simulink model "DCDC_SEPIC_ThermalModel"  (R2021b)
settings: Solver=VariableStepAuto  StartTime=0.0  StopTime=3600*24  RelTol=1e-3  EnableMultiTasking=on
undefined symbols (not defined in the file): Curr_Test_Load, Voltage_Test_Vector
libraries: fl_lib x19, nesl_utility x3
Description:
  | Buck Converter Thermal Model
settings Model: FPTRunName=Active  Creator=The MathWorks, Inc.  LastModifiedBy=vlenzi
settings SolverCC: AlgebraicLoopSolver=TrustRegion
settings DataIOCC: MaxDataPoints=10000  SaveFormat=Array  SaveOutput=off  SignalLogging=off  DSMLogging=off  SaveTime=off  SignalLoggingName=logsout_ee_switching_power_supply_thermal_only
settings OptimizationCC: BooleanDataType=off  ExpressionDepthLimit=2147483647  InitFltsAndDblsToZero=on  LifeSpan=1  EfficientTunableParamExpr=on
settings DebuggingCC: SaveWithParameterizedLinksMsg=none  SignalResolutionControl=TryResolveAllWithWarning  MultiTaskDSMMsg=warning  MultiTaskCondExecSysMsg=none  IntegerOverflowMsg=none  ParameterPrecisionLossMsg=none  StateNameClashWarn=warning  SFUnexpectedBacktrackingDiag=warning  SFNoUnconditionalDefaultTransitionDiag=warning  SFExecutionAtInitializationDiag=none  SFMachineParentedDataDiag=warning  IntegerSaturationMsg=none  ArithmeticOperatorsInVariantConditions=warning
settings HardwareCC: ProdBitPerPointer=32  ProdBitPerSizeT=32  ProdBitPerPtrDiffT=32  ProdLargestAtomicFloat=None  ProdIntDivRoundTo=Undefined  ProdEndianess=Unspecified  ProdWordSize=32  ProdHWDeviceType=32-bit Generic
settings ModelReferenceCC: PropagateSignalLabelsOutOfModel=off
settings SFSimCC: SimUseLocalCustomCode=off  CustomCodeUndefinedFunction=UseInterfaceOnly
settings RTWCC: Description=Real-Time Workshop Embedded Coder (no auto configuration)  SystemTargetFile=ert.tlc  TemplateMakefile=ert_default_tmf  GenerateReport=on  RTWUseLocalCustomCode=off  IncludeHyperlinkInReport=on  LaunchReport=on  CreateSILPILBlock=SIL
settings CodeAppCC: IgnoreCustomStorageClasses=off  CustomSymbolStrType=$N$R$M  CustomSymbolStrModelFcn=$N  StateflowObjectComments=on  InternalIdentifier=Classic
settings ERTTargetCC: TargetFcnLib=ansi_tfl_tmw.mat  MultiwordLength=2048  GenerateSampleERTMain=on  ERTCustomFileTemplate=example_file_process.tlc  ConvertIfToSwitch=off  SuppressUnreachableDefaultCases=off
settings ConfigComp: CovMetricSettings=dw  CovSaveCumulativeToWorkspaceVar=on  CovSaveSingleToWorkspaceVar=on  CovExternalEMLEnable=off  CovSFcnEnable=off
settings SimscapeCC: SimscapeLogType=all  SimscapeLogSimulationStatistics=on  SimscapeLogToSDI=on  SimscapeLogName=simlog_ee_switching_power_supply_thermal_only  SimscapeLogLimitData=off  SimscapeLogDataHistory=10000

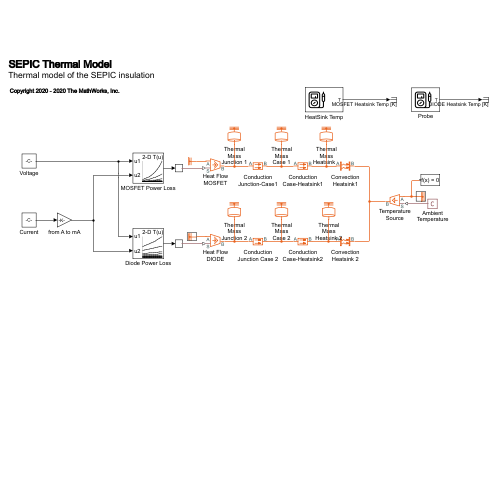
[thumbnail: Simulink's stored preview of the top-level diagram]
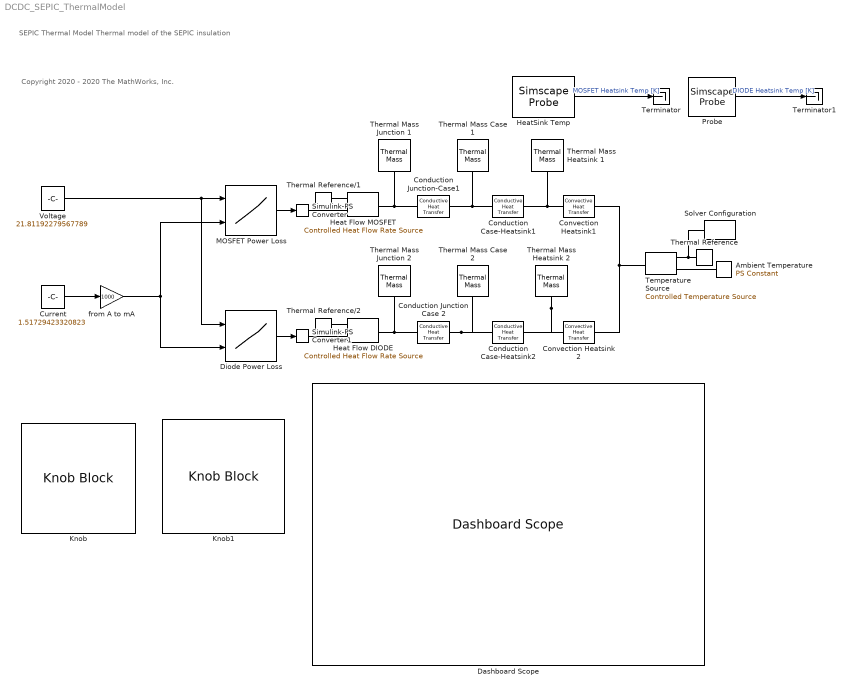
== system DCDC_SEPIC_ThermalModel ==
  note: SEPIC Thermal Model
      | Thermal model of the SEPIC insulation
  note: Copyright 2020 - 2020 The MathWorks, Inc.
  Ambient Temperature : fl_lib/Physical Signals/Sources/PS Constant  constant=298.15
  Conduction Case-Heatsink1 : fl_lib/Thermal/Thermal Elements/Conductive Heat Transfer  area=14 mm^2  thickness=0.1 mm  th_cond=3 W/(m*K)  T_specify=off  T_priority=High  T=0 K  T_nominal_specify=off  T_nominal_unit=K  T_nominal_value=1  Q_specify=off  Q_priority=High  Q=0 J/s  Q_nominal_specify=off  Q_nominal_unit=J/s  Q_nominal_value=1
  Conduction Case-Heatsink2 : fl_lib/Thermal/Thermal Elements/Conductive Heat Transfer  area=14 mm^2  thickness=0.1 mm  th_cond=3 W/(m*K)  T_specify=off  T_priority=High  T=0 K  T_nominal_specify=off  T_nominal_unit=K  T_nominal_value=1  Q_specify=off  Q_priority=High  Q=0 J/s  Q_nominal_specify=off  Q_nominal_unit=J/s  Q_nominal_value=1
  Conduction Junction Case 2 : fl_lib/Thermal/Thermal Elements/Conductive Heat Transfer  area=5 mm^2  thickness=360 um  th_cond=150 W/(m*K)  T_specify=off  T_priority=High  T=0 K  T_nominal_specify=off  T_nominal_unit=K  T_nominal_value=1  Q_specify=off  Q_priority=High  Q=0 J/s  Q_nominal_specify=off  Q_nominal_unit=J/s  Q_nominal_value=1
  Conduction Junction-Case1 : fl_lib/Thermal/Thermal Elements/Conductive Heat Transfer  area=5 mm^2  thickness=360 um  th_cond=150 W/(m*K)  T_specify=off  T_priority=High  T=0 K  T_nominal_specify=off  T_nominal_unit=K  T_nominal_value=1  Q_specify=off  Q_priority=High  Q=0 J/s  Q_nominal_specify=off  Q_nominal_unit=J/s  Q_nominal_value=1
  Convection Heatsink 2 : fl_lib/Thermal/Thermal Elements/Convective Heat Transfer  area=40 cm^2  heat_tr_coeff=20 W/(m^2 * K)  T_specify=off  T_priority=High  T=0 K  T_nominal_specify=off  T_nominal_unit=K  T_nominal_value=1  Q_specify=off  Q_priority=High  Q=0 J/s  Q_nominal_specify=off  Q_nominal_unit=J/s  Q_nominal_value=1
  Convection Heatsink1 : fl_lib/Thermal/Thermal Elements/Convective Heat Transfer  area=40 cm^2  heat_tr_coeff=20 W/(m^2 * K)  T_specify=off  T_priority=High  T=0 K  T_nominal_specify=off  T_nominal_unit=K  T_nominal_value=1  Q_specify=off  Q_priority=High  Q=0 J/s  Q_nominal_specify=off  Q_nominal_unit=J/s  Q_nominal_value=1
  Current : Constant  Value=1.51729423320823
  Dashboard Scope : DashboardScope  Ymin=273  Ymax=350
  Diode Power Loss : Lookup_n-D  BreakpointsForDimension1=Voltage_Test_Vector  BreakpointsForDimension2=Curr_Test_Load  Table=diodeLosses_grid'  ExtrapMethod=Clip  InternalRulePriority=Speed  RndMeth=Simplest  InputSameDT=on
      settings: InputPortMap=u0,u1
  Heat Flow DIODE : fl_lib/Thermal/Thermal Sources/Controlled Heat Flow Rate Source
  Heat Flow MOSFET : fl_lib/Thermal/Thermal Sources/Controlled Heat Flow Rate Source
  HeatSink Temp : SimscapeProbe  BoundBlock=254  Variables={T}
  Knob : KnobBlock  ScaleMin=10  ScaleMax=26
  Knob1 : KnobBlock  ScaleMax=2
  MOSFET Power Loss : Lookup_n-D  BreakpointsForDimension1=Voltage_Test_Vector  BreakpointsForDimension2=Curr_Test_Load  Table=mosfetLosses_grid'  InternalRulePriority=Speed  RndMeth=Simplest  InputSameDT=on
      settings: InputPortMap=u0,u1
  Probe : SimscapeProbe  BoundBlock=256  Variables={T}
  Simulink-PS Converter : nesl_utility/Simulink-PS Converter  PhysicalDomain=network_engine_domain  SubClassName=ps_input  LeftPortType=input  RightPortType=output  PseudoPeriodic=off  Frequencies=[]  NoiseDistribution=none  NoiseParameters=[]  Unit=J/s  AffineConversion=off  FilteringAndDerivatives=provide  SimscapeFilterOrder=1  InputFilterTimeConstant=0.001  UdotUserProvided=0
      settings: SourceProductBaseCode=PW,SS
  Simulink-PS Converter1 : nesl_utility/Simulink-PS Converter  PhysicalDomain=network_engine_domain  SubClassName=ps_input  LeftPortType=input  RightPortType=output  PseudoPeriodic=off  Frequencies=[]  NoiseDistribution=none  NoiseParameters=[]  Unit=J/s  AffineConversion=off  FilteringAndDerivatives=provide  SimscapeFilterOrder=1  InputFilterTimeConstant=0.001  UdotUserProvided=0
      settings: SourceProductBaseCode=PW,SS
  Solver Configuration : nesl_utility/Solver Configuration  PhysicalDomain=network_engine_domain  SubClassName=solver  LeftPortType=input  RightPortType=generic  Tones=[]  Harmonics=[]  SimulateNoise=off  Profile=off  UseLocalSampling=off  EnableSwitchedLinearOptims=on  FrequencyDomain=off  UseCCode=off  RelTol=0.001  AbsTol=1e-06  MinStep=1e-09  ToWorkspace=off  RevertToSquareIcSolve=off  NumHomotopyIterations=100  PhasorMode=off  PhasorModeNumHarmonics=1  DoDC=off  ResidualTolerance=1e-9  UseLocalSolver=off  LocalSolverChoice=NE_BACKWARD_EULER_ADVANCER  LocalSolverSampleTime=.001  DoFixedCost=off  MaxNonlinIter=12  MaxModeIter=2  ComputeImpulses=off  ImpulseIterations=2  LinearAlgebra=auto  EquationFormulation=NE_TIME_EF  DelaysMemoryBudget=1024  AutomaticFiltering=on  FilteringTimeConstant=0.001  PartitionStorageMethod=AS_NEEDED  PartitionMemoryBudget=1024  PartitionMethod=FAST
      settings: SourceProductBaseCode=PW,SS
  Temperature Source : fl_lib/Thermal/Thermal Sources/Controlled Temperature Source
  Terminator : Terminator
  Terminator1 : Terminator
  Thermal Mass Case 1 : fl_lib/Thermal/Thermal Elements/Thermal Mass  mass=0.8 g  sp_heat=385 J/kg/K  T_specify=on  T_priority=High  T=298.15 K  T_nominal_specify=off  T_nominal_unit=K  T_nominal_value=1  Q_specify=off  Q_priority=High  Q=0 J/s  Q_nominal_specify=off  Q_nominal_unit=J/s  Q_nominal_value=1
  Thermal Mass Case 2 : fl_lib/Thermal/Thermal Elements/Thermal Mass  mass=0.8 g  sp_heat=385 J/kg/K  T_specify=on  T_priority=High  T=298.15 K  T_nominal_specify=off  T_nominal_unit=K  T_nominal_value=1  Q_specify=off  Q_priority=High  Q=0 J/s  Q_nominal_specify=off  Q_nominal_unit=J/s  Q_nominal_value=1
  Thermal Mass Heatsink 1 : fl_lib/Thermal/Thermal Elements/Thermal Mass  mass=0.01 kg  sp_heat=900 J/kg/K  T_specify=on  T_priority=High  T=298.15 K  T_nominal_specify=off  T_nominal_unit=K  T_nominal_value=1  Q_specify=off  Q_priority=High  Q=0 J/s  Q_nominal_specify=off  Q_nominal_unit=J/s  Q_nominal_value=1
  Thermal Mass Heatsink 2 : fl_lib/Thermal/Thermal Elements/Thermal Mass  mass=0.01 kg  sp_heat=900 J/kg/K  T_specify=on  T_priority=High  T=298.15 K  T_nominal_specify=off  T_nominal_unit=K  T_nominal_value=1  Q_specify=off  Q_priority=High  Q=0 J/s  Q_nominal_specify=off  Q_nominal_unit=J/s  Q_nominal_value=1
  Thermal Mass Junction 1 : fl_lib/Thermal/Thermal Elements/Thermal Mass  mass=4.2 mg  sp_heat=700 J/kg/K  T_specify=on  T_priority=High  T=298.15 K  T_nominal_specify=off  T_nominal_unit=K  T_nominal_value=1  Q_specify=off  Q_priority=High  Q=0 J/s  Q_nominal_specify=off  Q_nominal_unit=J/s  Q_nominal_value=1
  Thermal Mass Junction 2 : fl_lib/Thermal/Thermal Elements/Thermal Mass  mass=4.2 mg  sp_heat=700 J/kg/K  T_specify=on  T_priority=High  T=298.15 K  T_nominal_specify=off  T_nominal_unit=K  T_nominal_value=1  Q_specify=off  Q_priority=High  Q=0 J/s  Q_nominal_specify=off  Q_nominal_unit=J/s  Q_nominal_value=1
  Thermal Reference/1 : fl_lib/Thermal/Thermal Elements/Thermal Reference
  Thermal Reference/2 : fl_lib/Thermal/Thermal Elements/Thermal Reference
  Thermal Reference : fl_lib/Thermal/Thermal Elements/Thermal Reference
  Voltage : Constant  Value=21.81192279567789
  from A to mA : Gain  Gain=1000
  wires:
  Voltage/1 -> Diode Power Loss/1, MOSFET Power Loss/1
  Current/1 -> from A to mA/1
  MOSFET Power Loss/1 -> Simulink-PS Converter/1
  Diode Power Loss/1 -> Simulink-PS Converter1/1
  from A to mA/1 -> Diode Power Loss/2, MOSFET Power Loss/2
  HeatSink Temp/1 -> Terminator/1  "MOSFET Heatsink Temp [K]"
  Probe/1 -> Terminator1/1  "DIODE Heatsink Temp [K]"
  connections:
  Conduction Case-Heatsink1/RConn1 -- Convection Heatsink1/LConn1 -- Thermal Mass Heatsink 1/LConn1
  Conduction Junction-Case1/LConn1 -- Heat Flow MOSFET/LConn1 -- Thermal Mass Junction 1/LConn1
  Conduction Case-Heatsink1/LConn1 -- Conduction Junction-Case1/RConn1 -- Thermal Mass Case 1/LConn1
  Thermal Reference/1/LConn1 -- Heat Flow MOSFET/RConn2
  Simulink-PS Converter/RConn1 -- Heat Flow MOSFET/RConn1
  Conduction Junction Case 2/LConn1 -- Heat Flow DIODE/LConn1 -- Thermal Mass Junction 2/LConn1
  Conduction Junction Case 2/RConn1 -- Conduction Case-Heatsink2/LConn1 -- Thermal Mass Case 2/LConn1
  Simulink-PS Converter1/RConn1 -- Heat Flow DIODE/RConn1
  Thermal Reference/2/LConn1 -- Heat Flow DIODE/RConn2
  Convection Heatsink 2/RConn1 -- Convection Heatsink1/RConn1 -- Temperature Source/LConn1
  Ambient Temperature/RConn1 -- Temperature Source/RConn1
  Thermal Reference/LConn1 -- Solver Configuration/RConn1 -- Temperature Source/RConn2
  Thermal Mass Heatsink 2/LConn1 -- Conduction Case-Heatsink2/RConn1 -- Convection Heatsink 2/LConn1
